simulink model "kinematic_bycicle"  (R2015b)
settings: Solver=VariableStepAuto  StartTime=0.0  StopTime=10.0  MaxStep=0.01  RelTol=1e-3
values from neighbouring files (symbols this model uses):
  Lf = 1    [KINEMATIC_MOTION_PLANNER.m]    (also in KINEMATIC_MOTION_PLANNER2.m; KINEMATIC_STEP_MPC.m; KINEMATIC_VEHICLE_CONTROL.m; KINEMATIC_VEHICLE_SIM.m)
  Lr = 1    [KINEMATIC_MOTION_PLANNER.m]    (also in KINEMATIC_MOTION_PLANNER2.m; KINEMATIC_STEP_MPC.m; KINEMATIC_VEHICLE_CONTROL.m; KINEMATIC_VEHICLE_SIM.m)
  Psi0 = 0    [KINEMATIC_MOTION_PLANNER.m]    (also in KINEMATIC_MOTION_PLANNER2.m; KINEMATIC_STEP_MPC.m; KINEMATIC_VEHICLE_CONTROL.m; KINEMATIC_VEHICLE_SIM.m)
  V = 1    [KINEMATIC_MOTION_PLANNER.m]    (also in KINEMATIC_MOTION_PLANNER2.m; KINEMATIC_STEP_MPC.m; KINEMATIC_VEHICLE_CONTROL.m; KINEMATIC_VEHICLE_SIM.m = 5)
  X0 = 0    [KINEMATIC_MOTION_PLANNER.m]    (also in KINEMATIC_MOTION_PLANNER2.m; KINEMATIC_STEP_MPC.m; KINEMATIC_VEHICLE_CONTROL.m; KINEMATIC_VEHICLE_SIM.m)
  Y0 = 0    [KINEMATIC_MOTION_PLANNER.m]    (also in KINEMATIC_MOTION_PLANNER2.m; KINEMATIC_STEP_MPC.m; KINEMATIC_VEHICLE_CONTROL.m; KINEMATIC_VEHICLE_SIM.m)
settings Model: Creator=gebruiker  LastModifiedBy=gebruiker

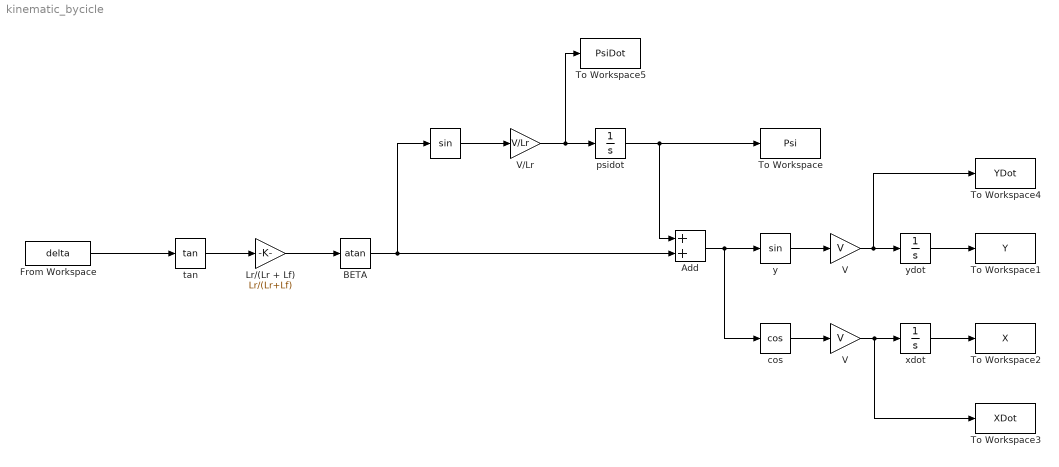
== system kinematic_bycicle ==
  " " : Trigonometry  OutputSignalType=real
  Add : Sum
  BETA : Trigonometry  Operator=atan  OutputSignalType=real
  From Workspace : FromWorkspace  VariableName=delta  SampleTime=0
  Lr/(Lr + Lf) : Gain  Gain=Lr/(Lr+Lf)
  To Workspace : ToWorkspace  VariableName=Psi  SaveFormat=Structure With Time  SampleTime=-1
  To Workspace1 : ToWorkspace  VariableName=Y  SaveFormat=Structure With Time  SampleTime=-1
  To Workspace2 : ToWorkspace  VariableName=X  SaveFormat=Structure With Time  SampleTime=-1
  To Workspace3 : ToWorkspace  VariableName=XDot  SaveFormat=Structure With Time  SampleTime=-1
  To Workspace4 : ToWorkspace  VariableName=YDot  SaveFormat=Structure With Time  SampleTime=-1
  To Workspace5 : ToWorkspace  VariableName=PsiDot  SaveFormat=Structure With Time  SampleTime=-1
  V : Gain  Gain=V
  "V " : Gain  Gain=V
  V/Lr : Gain  Gain=V/Lr
  cos : Trigonometry  Operator=cos  OutputSignalType=real
  psidot : Integrator  InitialCondition=Psi0
  "tan " : Trigonometry  Operator=tan  OutputSignalType=real
  xdot : Integrator  InitialCondition=X0
  y : Trigonometry  OutputSignalType=real
  ydot : Integrator  InitialCondition=Y0
  wires:
  "tan "/1 -> Lr/(Lr + Lf)/1
  Lr/(Lr + Lf)/1 -> BETA/1
  From Workspace/1 -> "tan "/1
  " "/1 -> V/Lr/1
  BETA/1 -> Add/2, " "/1
  V/Lr/1 -> To Workspace5/1, psidot/1
  psidot/1 -> Add/1, To Workspace/1
  y/1 -> V/1
  ydot/1 -> To Workspace1/1
  Add/1 -> cos/1, y/1
  cos/1 -> "V "/1
  "V "/1 -> To Workspace3/1, xdot/1
  xdot/1 -> To Workspace2/1
  V/1 -> To Workspace4/1, ydot/1
